simulink model "FSK_2023b"  (R2023b)
settings: Solver=VariableStepDiscrete  StartTime=0.0  StopTime=2000/Rb  RelTol=1e-3  EnableMultiTasking=on
PreLoadFcn:
  | fc=30000;
  | Rb=9600;
  | df=Rb;
libraries: commrandsrc2 x1
settings Model: Creator=morelos_zaragoza  LastModifiedBy=14083
settings SolverCC: AlgebraicLoopSolver=TrustRegion
settings DataIOCC: LimitDataPoints=on  SaveFormat=Array  SignalLoggingSaveFormat=ModelDataLogs  ReturnWorkspaceOutputs=off
settings OptimizationCC: ExpressionDepthLimit=2147483647  InitFltsAndDblsToZero=on  LifeSpan=inf
settings DebuggingCC: SaveWithParameterizedLinksMsg=none  UnderspecifiedInitializationDetection=Classic  MergeDetectMultiDrivingBlocksExec=none  SignalResolutionControl=TryResolveAllWithWarning  SolverPrmCheckMsg=warning  MultiTaskDSMMsg=warning  MultiTaskCondExecSysMsg=none  FcnCallInpInsideContextMsg=warning  UnconnectedInputMsg=warning  UnconnectedOutputMsg=warning  UnconnectedLineMsg=warning  StateNameClashWarn=warning  SFUnexpectedBacktrackingDiag=warning  SFNoUnconditionalDefaultTransitionDiag=warning  SFExecutionAtInitializationDiag=none  ArithmeticOperatorsInVariantConditions=warning
settings HardwareCC: ProdBitPerPointer=32  ProdBitPerSizeT=32  ProdBitPerPtrDiffT=32  ProdLargestAtomicFloat=None  ProdIntDivRoundTo=Undefined  ProdEndianess=Unspecified  ProdWordSize=32  ProdHWDeviceType=32-bit Generic
settings ModelReferenceCC: EnableRefExpFcnMdlSchedulingChecks=on  PropagateSignalLabelsOutOfModel=off
settings SFSimCC: SimUseLocalCustomCode=off  CustomCodeUndefinedFunction=UseInterfaceOnly
settings RTWCC: RTWUseLocalCustomCode=off
settings CodeAppCC: StateflowObjectComments=on
settings GRTTargetCC: TargetFcnLib=ansi_tfl_tmw.mat  TargetLangStandard=C89/C90 (ANSI)  CombineOutputUpdateFcns=off  GRTInterface=on
settings ConfigComp: CovMetricSettings=dw  CovSaveCumulativeToWorkspaceVar=on  CovSaveSingleToWorkspaceVar=on  CovExternalEMLEnable=off

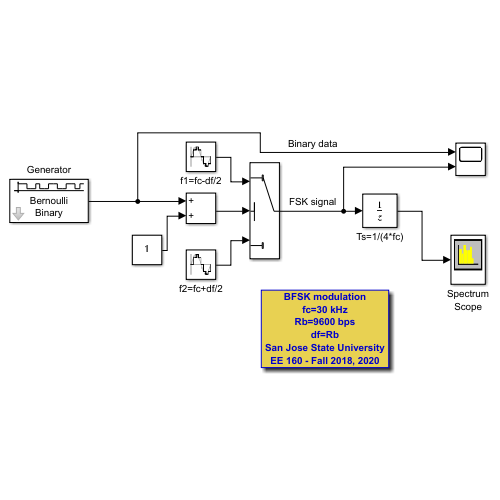
[thumbnail: Simulink's stored preview of the top-level diagram]
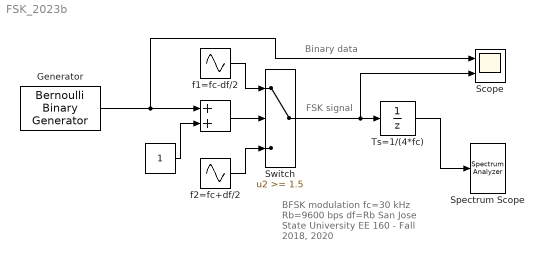
== system FSK_2023b ==
  note: FSK signal
  note: Binary data
  note: BFSK modulation
      | fc=30 kHz
      | Rb=9600 bps
      | df=Rb
      | San Jose State University
      | EE 160 - Fall 2018, 2020
  " " : Constant
  "  " : Sum
  Generator : commrandsrc2/Bernoulli Binary Generator  P=1/2  seed=seed  Ts=1/Rb  frameBased=off  sampPerFrame=1  orient=off  outDataType=double
  Scope : Scope  NumInputPorts=2
  Spectrum Scope : SpectrumAnalyzer  WindowPosition=[4.000000,34.000000,413.000000,386.000000,]  Visible=on  ScopeFrameLocation=window  Method=Welch  SampleRate=120000  PlotAsTwoSidedSpectrum=off  AxesScaling=Manual  Span=60000  CenterFrequency=30000  StartFrequency=0  StopFrequency=60000  FrequencyResolutionMethod=Window length  FFTLengthSource=Property  FFTLength=512  WindowLength=512  OverlapPercent=25  AveragingMethod=Running  SpectralAverages=100  YLabel=Magnitude  YLimits=[-15,25]  DefaultConfigurationName=spbscopes.SpectrumAnalyzerBlockCfg  IsFrequencyInputMode=0  FrequencyVectorPort=0  FrequencyVectorFromPort=0  FrequencyInputRBWPort=0  FrequencyInputRBWFromPort=0  SegLen=512
  Switch : Switch  Threshold=1.5  SaturateOnIntegerOverflow=off  InputSameDT=off
  Ts=1/(4*fc) : UnitDelay  SampleTime=1/(4*fc)  HasFrameUpgradeWarning=on
  f1=fc-df/2 : Sin  Frequency=2*pi*(fc-df/2)  SampleTime=1/(16*fc)
  f2=fc+df/2 : Sin  Frequency=2*pi*(fc+df/2)  SampleTime=1/(16*fc)
  wires:
  f1=fc-df/2/1 -> Switch/1
  f2=fc+df/2/1 -> Switch/3
  " "/1 -> "  "/2
  "  "/1 -> Switch/2
  Switch/1 -> Ts=1/(4*fc)/1, Scope/2
  Ts=1/(4*fc)/1 -> Spectrum Scope/1
  Generator/1 -> "  "/1, Scope/1
